simulink model "Copy_2_of_system2"  (R2019b)
settings: Solver=VariableStepAuto  StartTime=0.0  StopTime=15  RelTol=1e-5
Description:
  | 高阶系统闭环主导极点分析
settings Model: Creator=Inspiron  LastModifiedBy=Inspiron

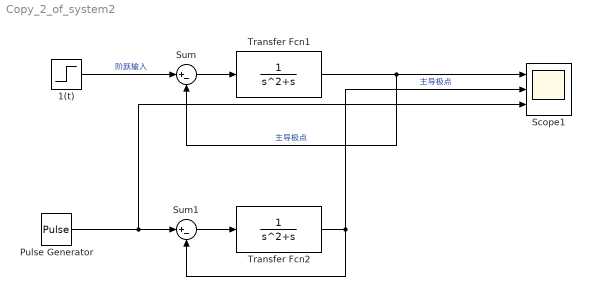
== system Copy_2_of_system2 ==
  1(t) : Step  Time=0  SampleTime=0
  Pulse Generator : DiscretePulseGenerator  PulseType=Time based  Amplitude=10000  Period=0.1  PulseWidth=0.01
  Scope1 : Scope  NumInputPorts=3
  Sum : Sum  Inputs=|+-
  Sum1 : Sum  Inputs=|+-
  Transfer Fcn1 : TransferFcn  Denominator=[1 1 0]
  Transfer Fcn2 : TransferFcn  Denominator=[1 1 0]
  wires:
  Transfer Fcn1/1 -> Scope1/1, Sum/2  "主导极点"
  1(t)/1 -> Sum/1  "阶跃输入"
  Sum/1 -> Transfer Fcn1/1
  Sum1/1 -> Transfer Fcn2/1
  Pulse Generator/1 -> Scope1/3, Sum1/1
  Transfer Fcn2/1 -> Scope1/2, Sum1/2  "主导极点"
